simulink model "fig9_22"  (Simulink 8.4)
settings: Solver=ode45  SolverMode=SingleTasking  StartTime=0.0  StopTime=10.0  RelTol=1e-3  AbsTol=1e-6
undefined symbols (not defined in the file or in its folder): ka
settings Model: Creator=abbas  LastModifiedBy=abbas  ExtModeTrigMode=oneshot  ExtModeArmWhenConnect=off
settings DataIOCC: LimitDataPoints=off
settings OptimizationCC: BlockReduction=off  BooleanDataType=off  InitFltsAndDblsToZero=on
settings DebuggingCC: SaveWithParameterizedLinksMsg=none  SignalResolutionControl=TryResolveAllWithWarning  SolverPrmCheckMsg=none  MultiTaskDSMMsg=warning  MultiTaskCondExecSysMsg=none
settings HardwareCC: TargetUnknown=on
settings RTWCC: IncludeERTFirstTime=on
settings GRTTargetCC: TargetFcnLib=ansi_tfl_tmw.mat  ModelReferenceCompliant=off  CompOptLevelCompliant=off  MatFileLogging=off

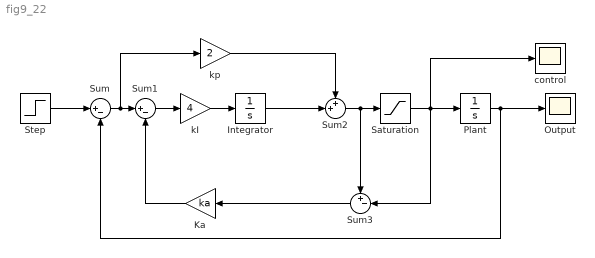
== system fig9_22 ==
  Integrator : Integrator
  Ka : Gain  Gain=ka  SaturateOnIntegerOverflow=on  OutDataTypeStr=Inherit: Same as input  ParamDataTypeStr=Inherit: Same as input
  Output : Scope
      settings: TickLabels=on  SaveName=yantib
  Plant : Integrator
  Saturation : Saturate  UpperLimit=1.0  LowerLimit=-1.0
  Step : Step  Time=.2  SampleTime=0.01
  Sum : Sum  Inputs=|+-  SaturateOnIntegerOverflow=on  InputSameDT=on  OutDataTypeStr=Inherit: Same as first input
  Sum1 : Sum  Inputs=|+-  SaturateOnIntegerOverflow=on  InputSameDT=on  OutDataTypeStr=Inherit: Same as first input
  Sum2 : Sum  Inputs=++|  SaturateOnIntegerOverflow=on  InputSameDT=on  OutDataTypeStr=Inherit: Same as first input
  Sum3 : Sum  Inputs=+-|  InputSameDT=on  OutDataTypeStr=Inherit: Same as first input
  control : Scope
      settings: TickLabels=on  SaveName=uantib
  kI : Gain  Gain=4  OutDataTypeStr=Inherit: Same as input  ParamDataTypeStr=Inherit: Same as input
  kp : Gain  Gain=2  OutDataTypeStr=Inherit: Same as input  ParamDataTypeStr=Inherit: Same as input
  wires:
  kI/1 -> Integrator/1
  Plant/1 -> Output/1, Sum/2
  Saturation/1 -> Plant/1, control/1, Sum3/2
  Sum1/1 -> kI/1
  Sum3/1 -> Ka/1
  Step/1 -> Sum/1
  Ka/1 -> Sum1/2
  Sum2/1 -> Saturation/1, Sum3/1
  Integrator/1 -> Sum2/2
  kp/1 -> Sum2/1
  Sum/1 -> Sum1/1, kp/1
